simulink model "feedback_harness"  (R2016a)
settings: Solver=ode45  StartTime=0.0  StopTime=4  RelTol=1e-3
settings Model: ModifiedByFormat=The MathWorks Inc.  Creator=The MathWorks, Inc.  LastModifiedBy=The MathWorks Inc.
settings DataIOCC: LimitDataPoints=on  SaveFormat=Array  SaveOutput=off  SaveTime=off
settings OptimizationCC: ExpressionDepthLimit=2147483647  LifeSpan=1
settings DebuggingCC: UnderspecifiedInitializationDetection=Classic  MergeDetectMultiDrivingBlocksExec=none  SolverPrmCheckMsg=warning  FcnCallInpInsideContextMsg=EnableAllAsWarning  StateNameClashWarn=warning
settings HardwareCC: ProdBitPerPointer=32  ProdLargestAtomicFloat=None  ProdIntDivRoundTo=Undefined  ProdEndianess=Unspecified  ProdWordSize=32  ProdHWDeviceType=32-bit Generic
settings ModelReferenceCC: PropagateSignalLabelsOutOfModel=off
settings GRTTargetCC: CombineOutputUpdateFcns=off  GRTInterface=on
settings ConfigComp: CovModelRefEnable=Off  CovSFcnEnable=off

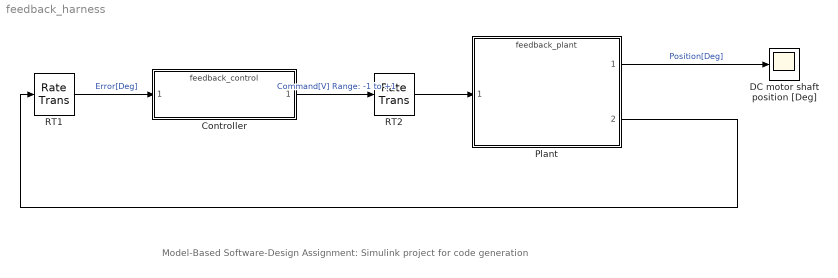
== system feedback_harness ==
  note: Model-Based Software-Design Assignment: Simulink project for code generation
  Controller : ModelReference  ModelNameDialog=feedback_control  SimulationMode=Normal  ModelReferenceVersion=1.42
  DC motor shaft position [Deg] : Scope
  Plant : ModelReference  ModelNameDialog=feedback_plant  SimulationMode=Normal  ModelReferenceVersion=1.28
  RT1 : RateTransition
  RT2 : RateTransition
  wires:
  Plant/2 -> RT1/1
  Controller/1 -> RT2/1  "Command[V] Range: -1 to +1"
  Plant/1 -> DC motor shaft position [Deg]/1  "Position[Deg]"
  RT1/1 -> Controller/1  "Error[Deg]"
  RT2/1 -> Plant/1
